simulink model "gm_gmStateSpaceHDL_uz_inverter_3ph"  (R2021b)
settings: Solver=FixedStepDiscrete  StartTime=0.0  StopTime=0.1  FixedStep=Auto  RelTol=1e-3
InitFcn:
  | load('C:\Users\valen\Documents\repos\UZ\ultrazohm_sw_working\ip_cores\uz_inverter_3ph\sschdl\uz_inverter_3ph\stateSpaceParameters.mat');
undefined symbols (not defined in the file or in its folder): udc
libraries: hdlmdlgenlib x140, dspsigops x26, simulink x17, hdlssclib x2
(part 1 of 2)
settings Model: Creator=LENOVO  LastModifiedBy=valen
settings SolverCC: AlgebraicLoopSolver=TrustRegion
settings DataIOCC: LimitDataPoints=on  SaveOutput=off  SaveTime=off
settings OptimizationCC: BlockReduction=off  ConditionallyExecuteInputs=off  DefaultParameterBehavior=Inlined  InheritOutputTypeSmallerThanSingle=on  LifeSpan=inf
settings DebuggingCC: AlgebraicLoopMsg=error  InheritedTsInSrcMsg=none  SingleTaskRateTransMsg=error  AllowSymbolicDim=off  StrictBusMsg=ErrorOnBusTreatedAsVector  SFUnexpectedBacktrackingDiag=warning  SFNoUnconditionalDefaultTransitionDiag=warning  SFExecutionAtInitializationDiag=none  SFMachineParentedDataDiag=warning  ArithmeticOperatorsInVariantConditions=warning
settings HardwareCC: ProdBitPerPointer=32  ProdBitPerSizeT=32  ProdBitPerPtrDiffT=32  ProdLargestAtomicFloat=None  ProdIntDivRoundTo=Undefined  ProdEndianess=Unspecified  ProdWordSize=32  ProdHWDeviceType=ASIC/FPGA->ASIC/FPGA  ProdEqTarget=off
settings SFSimCC: SimUseLocalCustomCode=off  CustomCodeUndefinedFunction=UseInterfaceOnly
settings RTWCC: RTWUseLocalCustomCode=off
settings CodeAppCC: StateflowObjectComments=on
settings GRTTargetCC: TargetLangStandard=C89/C90 (ANSI)
settings ConfigComp: CovScope=ReferencedModels  CovMetricSettings=dw  CovSaveCumulativeToWorkspaceVar=on  CovSaveSingleToWorkspaceVar=on  CovExternalEMLEnable=off  CovSFcnEnable=off

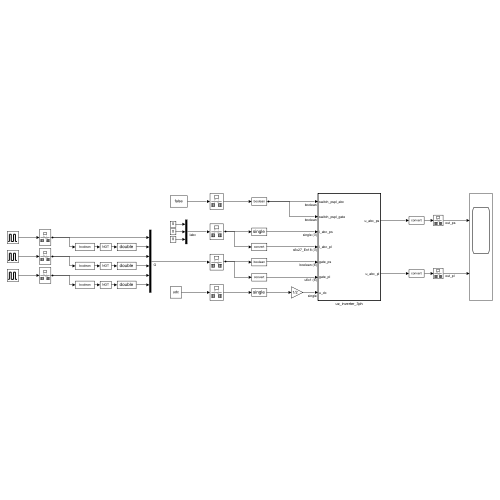
[thumbnail: Simulink's stored preview of the top-level diagram]
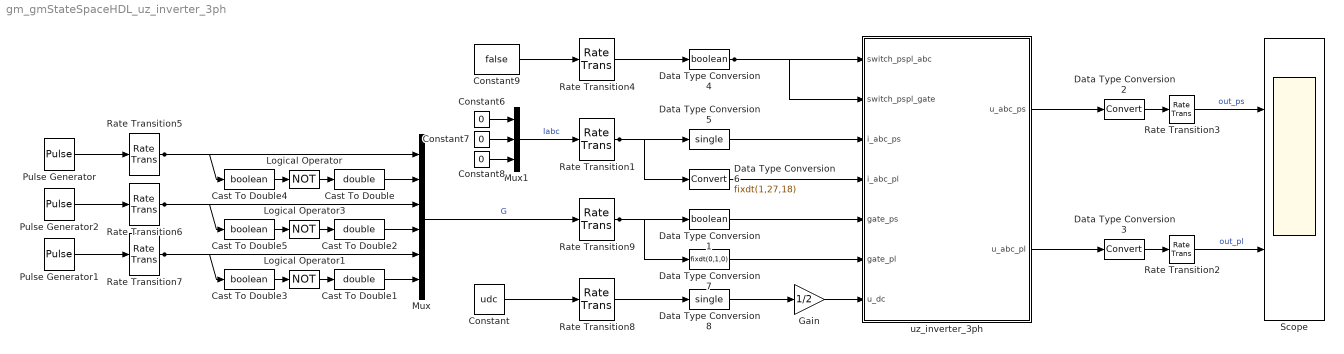
== system gm_gmStateSpaceHDL_uz_inverter_3ph ==
  Cast To Double : DataTypeConversion  OutDataTypeStr=double
  Cast To Double1 : DataTypeConversion  OutDataTypeStr=double
  Cast To Double2 : DataTypeConversion  OutDataTypeStr=double
  Cast To Double3 : DataTypeConversion  OutDataTypeStr=boolean
  Cast To Double4 : DataTypeConversion  OutDataTypeStr=boolean
  Cast To Double5 : DataTypeConversion  OutDataTypeStr=boolean
  Constant : Constant  Value=udc
  Constant6 : Constant  Value=0
  Constant7 : Constant  Value=0
  Constant8 : Constant  Value=0
  Constant9 : Constant  Value=false
  Data Type Conversion1 : DataTypeConversion  OutDataTypeStr=boolean  RndMeth=Nearest
  Data Type Conversion2 : DataTypeConversion
  Data Type Conversion3 : DataTypeConversion
  Data Type Conversion4 : DataTypeConversion  OutDataTypeStr=boolean
  Data Type Conversion5 : DataTypeConversion  OutDataTypeStr=single  RndMeth=Nearest
  Data Type Conversion6 : DataTypeConversion  OutDataTypeStr=fixdt(1,27,18)  RndMeth=Nearest
  Data Type Conversion7 : DataTypeConversion  OutDataTypeStr=fixdt(0,1,0)  RndMeth=Nearest
  Data Type Conversion8 : DataTypeConversion  OutDataTypeStr=single  RndMeth=Nearest
  Gain : Gain  Gain=1/2  OutDataTypeStr=Inherit: Same as input
  Logical Operator : Logic  Operator=NOT  AllPortsSameDT=off  OutDataTypeStr=boolean
  Logical Operator1 : Logic  Operator=NOT  AllPortsSameDT=off  OutDataTypeStr=boolean
  Logical Operator3 : Logic  Operator=NOT  AllPortsSameDT=off  OutDataTypeStr=boolean
  Mux : Mux  Inputs=6
  Mux1 : Mux  Inputs=3
  Pulse Generator : DiscretePulseGenerator  PulseType=Time based  Period=0.001  PulseWidth=50
  Pulse Generator1 : DiscretePulseGenerator  PulseType=Time based  Period=0.01  PulseWidth=50
  Pulse Generator2 : DiscretePulseGenerator  PulseType=Time based  Period=0.05  PulseWidth=50
  Rate Transition{1..9} (9 alike) : RateTransition  OutPortSampleTime=ts_inverter
  Scope : Scope  NumInputPorts=2
  uz_inverter_3ph : Subsystem  TreatAsAtomicUnit=on
  wires:
  Data Type Conversion4/1 -> uz_inverter_3ph/1(switch_pspl_abc), uz_inverter_3ph/2(switch_pspl_gate)
  Rate Transition5/1 -> Mux/1, Cast To Double4/1
  Rate Transition6/1 -> Mux/3, Cast To Double5/1
  Gain/1 -> uz_inverter_3ph/7(u_dc)
  Rate Transition8/1 -> Data Type Conversion8/1
  Constant/1 -> Rate Transition8/1
  Data Type Conversion8/1 -> Gain/1
  Rate Transition7/1 -> Mux/5, Cast To Double3/1
  Cast To Double/1 -> Mux/2
  Mux/1 -> Rate Transition9/1  "G"
  Logical Operator/1 -> Cast To Double/1
  Cast To Double1/1 -> Mux/6
  Cast To Double4/1 -> Logical Operator/1
  Cast To Double2/1 -> Mux/4
  Pulse Generator/1 -> Rate Transition5/1
  Pulse Generator2/1 -> Rate Transition6/1
  Logical Operator3/1 -> Cast To Double2/1
  Cast To Double5/1 -> Logical Operator3/1
  Pulse Generator1/1 -> Rate Transition7/1
  Cast To Double3/1 -> Logical Operator1/1
  Logical Operator1/1 -> Cast To Double1/1
  Data Type Conversion7/1 -> uz_inverter_3ph/6(gate_pl)
  Data Type Conversion5/1 -> uz_inverter_3ph/3(i_abc_ps)
  Data Type Conversion1/1 -> uz_inverter_3ph/5(gate_ps)
  Rate Transition9/1 -> Data Type Conversion1/1, Data Type Conversion7/1
  Data Type Conversion6/1 -> uz_inverter_3ph/4(i_abc_pl)
  Rate Transition1/1 -> Data Type Conversion6/1, Data Type Conversion5/1
  Constant7/1 -> Mux1/2
  Constant6/1 -> Mux1/1
  Constant8/1 -> Mux1/3
  Mux1/1 -> Rate Transition1/1  "Iabc"
  Rate Transition4/1 -> Data Type Conversion4/1
  Constant9/1 -> Rate Transition4/1
  Rate Transition2/1 -> Scope/2  "out_pl"
  Rate Transition3/1 -> Scope/1  "out_ps"
  Data Type Conversion2/1 -> Rate Transition3/1
  Data Type Conversion3/1 -> Rate Transition2/1
  uz_inverter_3ph/2(u_abc_pl) -> Data Type Conversion3/1
  uz_inverter_3ph/1(u_abc_ps) -> Data Type Conversion2/1

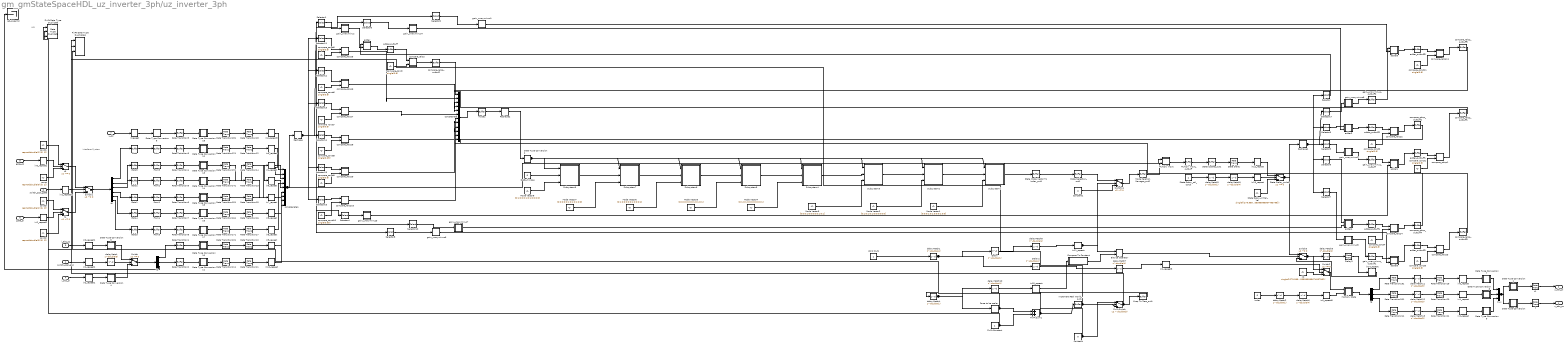
== system gm_gmStateSpaceHDL_uz_inverter_3ph/uz_inverter_3ph ==
  note: U(k)
  note: Interface System
  switch_pspl_abc : Inport  OutDataTypeStr=boolean  PortDimensions=1  SampleTime=1e-06
  switch_pspl_gate : Inport  Port=2  OutDataTypeStr=boolean  PortDimensions=1  SampleTime=1e-06
  i_abc_ps : Inport  Port=3  OutDataTypeStr=single  PortDimensions=[3]  SampleTime=1e-06
  i_abc_pl : Inport  Port=4  OutDataTypeStr=fixdt(1, 27, 18)  PortDimensions=[3]  SampleTime=1e-06
  gate_ps : Inport  Port=5  OutDataTypeStr=boolean  PortDimensions=[6]  SampleTime=1e-06  LockScale=on
  gate_pl : Inport  Port=6  OutDataTypeStr=fixdt(0, 1, 0)  PortDimensions=[6]  SampleTime=1e-06  LockScale=on
  u_dc : Inport  Port=7  OutDataTypeStr=single  PortDimensions=1  SampleTime=1e-06
  Bitwise Operator : simulink/Logic and Bit Operations/Bitwise Operator  logicop=AND  UseBitMask=off  NumInputPorts=2  BitMask=double(0)  BitMaskRealWorld=Real World Value
  Compare To Constant : Subsystem  mask(Compare To Constant){relop===, const=double(0), OutDataTypeStr=boolean, ZeroCross=on}
      mask prompts: relop "Simulink:masks:Operator_MP"; const "Simulink:masks:ConstantValue_MP"; OutDataTypeStr "Simulink:masks:OutputDataType_MP"; ZeroCross "Simulink:masks:EnableZerocrossingDetection_MP"
      mask help: Simulink:masks:CompareToConstant_MD
      mask TypeOptions relop: == | ~= | < | <= | >= | >
      mask TypeOptions OutDataTypeStr: Simulink:masks:uint8 | Simulink:masks:boolean
      mask Callback ZeroCross: sl('zeroCrossEnable', gcbh);
      mask Display: disp(str)
  Constant : Constant  Value=0  OutDataTypeStr=uint8  SampleTime=2.5e-07
  Constant1 : Constant  Value=0  OutDataTypeStr=fixdt(0, 3, 0)  SampleTime=1e-08
  Data Type Conversion : Subsystem
      mask Display: disp('NFP\nconv');
  Data Type Conversion1 : Subsystem
      mask Display: disp('NFP\nconv');
  Data Type Conversion10 : Subsystem
      mask Display: disp('NFP\nconv');
  Data Type Conversion11 : Subsystem
      mask Display: disp('NFP\nconv');
  Data Type Conversion12 : Subsystem
      mask Display: disp('NFP\nconv');
  Data Type Conversion13 : Subsystem
      mask Display: disp('NFP\nconv');
  Data Type Conversion14 : Subsystem
      mask Display: disp('NFP\nconv');
  Data Type Conversion15 : Subsystem
      mask Display: disp('NFP\nconv');
  Data Type Conversion16 : Subsystem
      mask Display: disp('NFP\nconv');
  Data Type Conversion17 : Subsystem
      mask Display: disp('NFP\nconv');
  Data Type Conversion18 : Subsystem
      mask Display: disp('NFP\nconv');
  Data Type Conversion2 : DataTypeConversion  OutDataTypeStr=boolean  SampleTime=1e-08
  Data Type Conversion3 : Subsystem
      mask Display: disp('NFP\nconv');
  Data Type Conversion4 : Subsystem
      mask Display: disp('NFP\nconv');
  Data Type Conversion6 : Subsystem
      mask Display: disp('NFP\nconv');
  Data Type Conversion7 : Subsystem
      mask Display: disp('NFP\nconv');
  Data Type Conversion8 : Subsystem
      mask Display: disp('NFP\nconv');
  Data Type Conversion9 : Subsystem
      mask Display: disp('NFP\nconv');
  Default Index : Constant  Value=0  OutDataTypeStr=fixdt(0, 3, 0)  SampleTime=1e-08
  Delay : Delay  DelayLength=double(1)  InitialCondition=0  SampleTime=2.5e-07
  Delay2 : Delay  DelayLength=double(4)  InitialCondition=0  SampleTime=2.5e-07
  Delay3 : RateTransition  OutPortSampleTimeOpt=Multiple of input port sample time  OutPortSampleTimeMultiple=25
  FixPt Constant : Constant  OutDataTypeStr=uint8  SampleTime=2.5e-07
  FixPt Data Type Duplicate : DataTypeDuplicate  DisableCoverage=on  NumInputPorts=3
  FixPt Data Type Duplicate1 : DataTypeDuplicate  DisableCoverage=on  NumInputPorts=3
  FixPt Sum1 : Sum  AccumDataTypeStr=uint8  OutDataTypeStr=uint8  SampleTime=2.5e-07
  FixPt Switch : Switch  Criteria=u2 > Threshold  Threshold=double(3)  OutDataTypeStr=uint8  SampleTime=2.5e-07
  Force to be scalar : SignalSpecification  OutDataTypeStr=uint8  Dimensions=1
  From{,1..5} (6 alike) : hdlmdlgenlib/Buffer
      settings: SourceProductBaseCode=SL
  Goto{,1..5} (6 alike) : hdlmdlgenlib/Buffer
      settings: SourceProductBaseCode=SL
  Iab_2_term2 : Terminator
  Increment Real World_out1 : hdlmdlgenlib/Buffer
      settings: SourceProductBaseCode=SL
  Index : Constant  Value=0  OutDataTypeStr=fixdt(0, 1, 0)  SampleTime=2.5e-07
  Mode Iteration Manager_out2 : hdlmdlgenlib/Buffer
      settings: SourceProductBaseCode=SL
  Mode Selection_out1 : hdlmdlgenlib/Buffer
      settings: SourceProductBaseCode=SL
  Mode Vector1 : Constant  Value=[0;0;0;1;0;1;0;0;0;1;0;0]  OutDataTypeStr=boolean  SampleTime=1e-08
  Mode Vector2 : Constant  Value=[0;1;0;1;0;1;0;0;0;0;0;0]  OutDataTypeStr=boolean  SampleTime=1e-08
  Mode Vector3 : Constant  Value=[0;0;0;1;0;0;0;0;0;1;0;1]  OutDataTypeStr=boolean  SampleTime=1e-08
  Mode Vector4 : Constant  Value=[0;1;0;1;0;0;0;0;0;0;0;1]  OutDataTypeStr=boolean  SampleTime=1e-08
  Mode Vector5 : Constant  Value=[0;0;0;0;0;0;0;1;0;1;0;1]  OutDataTypeStr=boolean  SampleTime=1e-08
  Mode Vector6 : Constant  Value=[0;1;0;0;0;0;0;1;0;0;0;1]  OutDataTypeStr=boolean  SampleTime=1e-08
  Mode Vector7 : Constant  Value=[0;0;0;0;0;1;0;1;0;1;0;0]  OutDataTypeStr=boolean  SampleTime=1e-08
  Mode Vector8 : Constant  Value=[0;1;0;0;0;1;0;1;0;0;0;0]  OutDataTypeStr=boolean  SampleTime=1e-08
  Multiply Input : Subsystem
      mask Display: disp('NFP\nSparseConstMultiply');
  Multiply Input_outbuff : hdlmdlgenlib/Buffer
      settings: SourceProductBaseCode=SL
  Multiply State : Subsystem
      mask Display: disp('NFP\nSparseConstMultiply');
  Rate Transition{1..9} (9 alike) : hdlmdlgenlib/Buffer
      settings: SourceProductBaseCode=SL
  Rate Transition{10..18} (9 alike) : RateTransition  Integrity=off  Deterministic=off  InitialCondition=double(0)  OutPortSampleTimeOpt=Multiple of input port sample time  OutPortSampleTimeMultiple=1/4
  Rate Transition{101,111,121,131,141,151,161,171,181} (9 alike) : RateTransition  OutPortSampleTimeOpt=Multiple of input port sample time  OutPortSampleTimeMultiple=100
  Rate Transition19 : RateTransition  InitialCondition=double(0)  OutPortSampleTimeOpt=Multiple of input port sample time  OutPortSampleTimeMultiple=4
  Rate Transition191 : RateTransition  OutPortSampleTimeOpt=Multiple of input port sample time  OutPortSampleTimeMultiple=25
  Rate Transition20 : RateTransition  InitialCondition=double(0)  OutPortSampleTimeOpt=Multiple of input port sample time  OutPortSampleTimeMultiple=4
  Rate Transition201 : RateTransition  OutPortSampleTimeOpt=Multiple of input port sample time  OutPortSampleTimeMultiple=25
  Rate Transition21 : RateTransition  InitialCondition=double(0)  OutPortSampleTimeOpt=Multiple of input port sample time  OutPortSampleTimeMultiple=4
  Rate Transition211 : RateTransition  OutPortSampleTimeOpt=Multiple of input port sample time  OutPortSampleTimeMultiple=25
  Reshape : Reshape  OutputDimensionality=Column vector (2-D)
  Reshape1 : Reshape  OutputDimensionality=Column vector (2-D)
  Reshape2 : Reshape
  Selector{,1..2,4,6..8,10} (8 alike) : Selector  SampleTime=1e-08  IndexOptions=Index vector (dialog)  Indices=double(1)  OutputSizes=double(0)
  Selector11 : Selector  SampleTime=1e-08  IndexOptions=Index vector (dialog)  Indices=double(2)  OutputSizes=double(0)
  Selector12 : Selector  SampleTime=1e-08  IndexOptions=Index vector (dialog)  Indices=double(3)  OutputSizes=double(0)
  Selector13 : Selector  SampleTime=1e-08  IndexOptions=Index vector (dialog)  Indices=double(4)  OutputSizes=double(0)
  Selector14 : Selector  SampleTime=1e-08  IndexOptions=Index vector (dialog)  Indices=double(5)  OutputSizes=double(0)
  Selector15 : Selector  SampleTime=1e-08  IndexOptions=Index vector (dialog)  Indices=double(6)  OutputSizes=double(0)
  Selector16 : Selector  SampleTime=1e-08  IndexOptions=Index vector (dialog)  Indices=double(7)  OutputSizes=double(0)
  Selector17 : Selector  SampleTime=1e-08  IndexOptions=Index vector (dialog)  Indices=double(2)  OutputSizes=double(0)
  Selector3 : Selector  SampleTime=1e-08  IndexOptions=Index vector (dialog)  Indices=double(3)  OutputSizes=double(0)
  Selector5 : Selector  SampleTime=1e-08  IndexOptions=Index vector (dialog)  Indices=double(2)  OutputSizes=double(0)
  Selector9 : Selector  SampleTime=1e-08  IndexOptions=Index vector (dialog)  Indices=double(3)  OutputSizes=double(0)
  State Delay : RateTransition  OutPortSampleTimeOpt=Multiple of input port sample time  OutPortSampleTimeMultiple=25
  State Delay_Initial_Val : Constant  Value=single([-279.99993896484375 -279.99993896484375 -279.99993896484375 -6.159998622301543e-10 0.0061599984765052795 -0.005599999334663153 0.0005599999567493796 -6.159998622301543e-10 0.0061599984765052795 0.0005599999567493796 0.0061599984765052795 0.0005599999567493796]).'  OutDataTypeStr=single  SampleTime=1e-08
  State Delay_ctrl_const : Constant  OutDataTypeStr=boolean  SampleTime=2.5e-07
  State Delay_switch : Switch  Criteria=u2 ~= 0  Threshold=double(0)  OutDataTypeStr=single  SampleTime=1e-08
  State Mode Vector To Index_out1 : hdlmdlgenlib/Buffer
      settings: SourceProductBaseCode=SL
  State Update_out1 : hdlmdlgenlib/Buffer
      settings: SourceProductBaseCode=SL
  Subsystem1 : Subsystem  mask{Index=fi(0,0,3,0,"hex","0")}
  Subsystem2 : Subsystem  mask{Index=fi(0,0,3,0,"hex","1")}
  Subsystem3 : Subsystem  mask{Index=fi(0,0,3,0,"hex","2")}
  Subsystem4 : Subsystem  mask{Index=fi(0,0,3,0,"hex","3")}
  Subsystem5 : Subsystem  mask{Index=fi(0,0,3,0,"hex","4")}
  Subsystem6 : Subsystem  mask{Index=fi(0,0,3,0,"hex","5")}
  Subsystem7 : Subsystem  mask{Index=fi(0,0,3,0,"hex","6")}
  Subsystem8 : Subsystem  mask{Index=fi(0,0,3,0,"hex","7")}
  Switch : Switch  Criteria=u2 ~= 0  Threshold=double(0)  OutDataTypeStr=double  SampleTime=1e-08
  Switch1 : Switch  Criteria=u2 ~= 0  Threshold=double(0)  OutDataTypeStr=double  SampleTime=1e-08
  Switch11 : Switch  Criteria=u2 ~= 0  Threshold=double(0)  OutDataTypeStr=fixdt(0, 3, 0)  SampleTime=1e-08
  Switch2 : Switch  Criteria=u2 ~= 0  Threshold=double(0)  OutDataTypeStr=single  SampleTime=1e-08
  Switch3 : Switch  Criteria=u2 ~= 0  Threshold=double(0)  OutDataTypeStr=single  SampleTime=1e-08
  Valid Out1 : Constant  OutDataTypeStr=boolean  SampleTime=2.5e-07
  Wrap To Zero_out1 : hdlmdlgenlib/Buffer
      settings: SourceProductBaseCode=SL
  X0 : Constant  Value=single([-279.99993896484375 -279.99993896484375 -279.99993896484375 -6.159998622301543e-10 0.0061599984765052795 -0.005599999334663153 0.0005599999567493796 -6.159998622301543e-10 0.0061599984765052795 0.0005599999567493796 0.0061599984765052795 0.0005599999567493796]).'  OutDataTypeStr=single  SampleTime=1e-08
  adder : Subsystem
      mask Display: disp('NFP\nadd');
  adder1 : Subsystem
      mask Display: disp('NFP\nadd');
  adder2 : Subsystem
      mask Display: disp('NFP\nadd');
  adder3 : Subsystem
      mask Display: disp('NFP\nadd');
  adder4 : Subsystem
      mask Display: disp('NFP\nadd');
  adder5 : Subsystem
      mask Display: disp('NFP\nadd');
  adder_outbuff{,1..5} (6 alike) : hdlmdlgenlib/Buffer
      settings: SourceProductBaseCode=SL
  compare_const{,1..4,11} (6 alike) : Constant  Value=single(0.8)  OutDataTypeStr=single  SampleTime=1e-08
  compare_const10 : Constant  Value=single(0.05)  OutDataTypeStr=single  SampleTime=1e-08
  compare_const{5..7,9} (4 alike) : Constant  Value=single(0.5)  OutDataTypeStr=single  SampleTime=1e-08
  compare_const8 : Constant  Value=single(0.05)  OutDataTypeStr=single  SampleTime=1e-08
  compare_relop : Subsystem
      mask Display: disp('NFP\nrelop');
  compare_relop1 : Subsystem
      mask Display: disp('NFP\nrelop');
  compare_relop10 : Subsystem
      mask Display: disp('NFP\nrelop');
  compare_relop11 : Subsystem
      mask Display: disp('NFP\nrelop');
  compare_relop2 : Subsystem
      mask Display: disp('NFP\nrelop');
  compare_relop3 : Subsystem
      mask Display: disp('NFP\nrelop');
  compare_relop4 : Subsystem
      mask Display: disp('NFP\nrelop');
  compare_relop5 : Subsystem
      mask Display: disp('NFP\nrelop');
  compare_relop6 : Subsystem
      mask Display: disp('NFP\nrelop');
  compare_relop7 : Subsystem
      mask Display: disp('NFP\nrelop');
  compare_relop8 : Subsystem
      mask Display: disp('NFP\nrelop');
  compare_relop9 : Subsystem
      mask Display: disp('NFP\nrelop');
  compare_relop_outbuff{,1..5} (6 alike) : hdlmdlgenlib/Buffer
      settings: SourceProductBaseCode=SL
  concatenate : Concatenate  NumInputs=12  ConcatenateDimension=2
  concatenate1 : Concatenate  NumInputs=9
  const : Constant  Value="repmat(double(0),[6  1])"  OutDataTypeStr=double  SampleTime=1e-08
  const1 : Constant  Value="repmat(double(1),[6  1])"  OutDataTypeStr=double  SampleTime=1e-08
  const2 : Constant  Value="repmat(double(0),[6  1])"  OutDataTypeStr=double  SampleTime=1e-08
  const3 : Constant  Value="repmat(double(1),[6  1])"  OutDataTypeStr=double  SampleTime=1e-08
  delayMatch : Delay  DelayLength=double(3)  InitialCondition=0  SampleTime=1e-08
  delayMatch{1,6..10} (6 alike) : Delay  DelayLength=double(4)  InitialCondition=0  SampleTime=2.5e-07
  delayMatch11 : Delay  DelayLength=double(3)  InitialCondition=0  SampleTime=2.5e-07
  delayMatch12 : Delay  DelayLength=double(3)  InitialCondition=0  SampleTime=2.5e-07
  delayMatch13 : Delay  DelayLength=double(3)  InitialCondition=0  SampleTime=2.5e-07
  delayMatch2 : Delay  DelayLength=double(1)  InitialCondition=0  SampleTime=2.5e-07
  delayMatch3 : Delay  DelayLength=double(1)  InitialCondition=0  SampleTime=2.5e-07
  delayMatch4 : Delay  DelayLength=double(1)  InitialCondition=0  SampleTime=2.5e-07
  delayMatch5 : Delay  DelayLength=double(1)  InitialCondition=0  SampleTime=1e-08
  gain_unaryminus : Subsystem
      mask Display: disp('NFP\numinus');
  gain_unaryminus1 : Subsystem
      mask Display: disp('NFP\numinus');
  gain_unaryminus2 : Subsystem
      mask Display: disp('NFP\numinus');
  gain_unaryminus3 : Subsystem
      mask Display: disp('NFP\numinus');
  gain_unaryminus4 : Subsystem
      mask Display: disp('NFP\numinus');
  gain_unaryminus5 : Subsystem
      mask Display: disp('NFP\numinus');
  gain_unaryminus6 : Subsystem
      mask Display: disp('NFP\numinus');
  gain_unaryminus7 : Subsystem
      mask Display: disp('NFP\numinus');
  gain_unaryminus8 : Subsystem
      mask Display: disp('NFP\numinus');
  gain_unaryminus_outbuff : hdlmdlgenlib/Buffer
      settings: SourceProductBaseCode=SL
  gain_unaryminus_outbuff1 : hdlmdlgenlib/Buffer
      settings: SourceProductBaseCode=SL
  gain_unaryminus_outbuff2 : hdlmdlgenlib/Buffer
      settings: SourceProductBaseCode=SL
  in0_repeat : dspsigops/Repeat  N=double(100)  RateOptions=Allow multirate processing  ic=0  mode=Unused parameter value
  in0_repeat1 : dspsigops/Repeat  N=double(100)  RateOptions=Allow multirate processing  ic=0  mode=Unused parameter value
  in0_repeat2 : dspsigops/Repeat  N=double(100)  RateOptions=Allow multirate processing  ic=0  mode=Unused parameter value
  in0_repeat3 : dspsigops/Repeat  N=double(25)  RateOptions=Allow multirate processing  ic=0  mode=Unused parameter value
  in10_repeat : dspsigops/Repeat  N=double(25)  RateOptions=Allow multirate processing  ic=0  mode=Unused parameter value
  in11_repeat : dspsigops/Repeat  N=double(25)  RateOptions=Allow multirate processing  ic=0  mode=Unused parameter value
  in12_repeat : dspsigops/Repeat  N=double(25)  RateOptions=Allow multirate processing  ic=0  mode=Unused parameter value
  in13_repeat : dspsigops/Repeat  N=double(25)  RateOptions=Allow multirate processing  ic=0  mode=Unused parameter value
  in14_repeat : dspsigops/Repeat  N=double(25)  RateOptions=Allow multirate processing  ic=0  mode=Unused parameter value
  in15_repeat : dspsigops/Repeat  N=double(25)  RateOptions=Allow multirate processing  ic=0  mode=Unused parameter value
  in1_repeat : dspsigops/Repeat  N=double(100)  RateOptions=Allow multirate processing  ic=0  mode=Unused parameter value
  in1_repeat1 : dspsigops/Repeat  N=double(100)  RateOptions=Allow multirate processing  ic=0  mode=Unused parameter value
  in1_repeat2 : dspsigops/Repeat  N=double(100)  RateOptions=Allow multirate processing  ic=0  mode=Unused parameter value
  in1_repeat3 : dspsigops/Repeat  N=double(25)  RateOptions=Allow multirate processing  ic=0  mode=Unused parameter value
  in2_repeat : dspsigops/Repeat  N=double(100)  RateOptions=Allow multirate processing  ic=0  mode=Unused parameter value
  in2_repeat1 : dspsigops/Repeat  N=double(100)  RateOptions=Allow multirate processing  ic=0  mode=Unused parameter value
  in2_repeat2 : dspsigops/Repeat  N=double(100)  RateOptions=Allow multirate processing  ic=0  mode=Unused parameter value
  in2_repeat3 : dspsigops/Repeat  N=double(25)  RateOptions=Allow multirate processing  ic=0  mode=Unused parameter value
  in3_repeat : dspsigops/Repeat  N=double(25)  RateOptions=Allow multirate processing  ic=0  mode=Unused parameter value
  in4_repeat : dspsigops/Repeat  N=double(25)  RateOptions=Allow multirate processing  ic=0  mode=Unused parameter value
  in5_repeat : dspsigops/Repeat  N=double(25)  RateOptions=Allow multirate processing  ic=0  mode=Unused parameter value
  in6_repeat : dspsigops/Repeat  N=double(25)  RateOptions=Allow multirate processing  ic=0  mode=Unused parameter value
  in7_repeat : dspsigops/Repeat  N=double(25)  RateOptions=Allow multirate processing  ic=0  mode=Unused parameter value
  in8_repeat : dspsigops/Repeat  N=double(25)  RateOptions=Allow multirate processing  ic=0  mode=Unused parameter value
  in9_repeat : dspsigops/Repeat  N=double(25)  RateOptions=Allow multirate processing  ic=0  mode=Unused parameter value
  inrepeat : dspsigops/Repeat  N=double(100)  RateOptions=Allow multirate processing  ic=0  mode=Unused parameter value
  modes : hdlmdlgenlib/Buffer
      settings: SourceProductBaseCode=SL
  mux : Mux  Inputs=3
  t : RateTransition  OutPortSampleTimeOpt=Multiple of input port sample time  OutPortSampleTimeMultiple=100
  t1 : RateTransition  OutPortSampleTimeOpt=Multiple of input port sample time  OutPortSampleTimeMultiple=100
  t2 : Demux  Outputs=3
  t3 : Switch  Criteria=u2 ~= 0  Threshold=double(0)  OutDataTypeStr=double  SampleTime=1e-08
  t4 : Switch  Criteria=u2 ~= 0  Threshold=double(0)  OutDataTypeStr=double  SampleTime=1e-08
  t5 : Demux  Outputs=6
  t6 : Demux  Outputs=3
  u_abc_ps : Outport  SampleTime=1e-06
  u_abc_pl : Outport  Port=2  SampleTime=1e-06
  wires:
  switch_pspl_abc/1 -> in1_repeat1/1
  switch_pspl_gate/1 -> in1_repeat2/1
  i_abc_ps/1 -> in0_repeat1/1
  i_abc_pl/1 -> in2_repeat1/1
  gate_ps/1 -> in0_repeat2/1
  gate_pl/1 -> in2_repeat2/1
  u_dc/1 -> inrepeat/1
  Rate Transition10/1 -> in9_repeat/1
  Rate Transition11/1 -> in10_repeat/1
  Rate Transition12/1 -> in3_repeat/1
  Rate Transition13/1 -> in7_repeat/1
  Rate Transition14/1 -> in6_repeat/1
  Rate Transition15/1 -> in4_repeat/1
  Rate Transition16/1 -> in8_repeat/1
  Rate Transition17/1 -> in5_repeat/1
  Rate Transition18/1 -> in2_repeat3/1
  Rate Transition19/1 -> in0_repeat/1
  Rate Transition20/1 -> in1_repeat/1
  Rate Transition21/1 -> in2_repeat/1
  delayMatch6/1 -> in0_repeat3/1
  delayMatch8/1 -> in11_repeat/1
  delayMatch7/1 -> in1_repeat3/1
  delayMatch1/1 -> Delay2/1, Delay/1
  delayMatch10/1 -> in15_repeat/1
  delayMatch9/1 -> in13_repeat/1
  delayMatch11/1 -> Rate Transition19/1
  delayMatch12/1 -> Rate Transition20/1
  delayMatch13/1 -> Rate Transition21/1
  t/1 -> u_abc_ps/1
  t1/1 -> u_abc_pl/1
  Rate Transition101/1 -> Rate Transition10/1
  Rate Transition111/1 -> Rate Transition11/1
  Rate Transition121/1 -> Rate Transition12/1
  Rate Transition131/1 -> Rate Transition13/1
  Rate Transition141/1 -> Rate Transition14/1
  Rate Transition151/1 -> Rate Transition15/1
  Rate Transition161/1 -> Rate Transition16/1
  Rate Transition171/1 -> Rate Transition17/1
  Rate Transition181/1 -> Rate Transition18/1
  delayMatch2/1 -> delayMatch6/1
  Delay2/1 -> delayMatch7/1
  Delay/1 -> delayMatch8/1
  delayMatch3/1 -> delayMatch9/1
  delayMatch4/1 -> delayMatch10/1, Force to be scalar/1
  Delay3/1 -> in14_repeat/1
  State Delay/1 -> in12_repeat/1
  Rate Transition191/1 -> delayMatch11/1
  Rate Transition201/1 -> delayMatch12/1
  Rate Transition211/1 -> delayMatch13/1
  Data Type Conversion/1(Out1) -> t/1
  Data Type Conversion1/1(Out1) -> t1/1
  in0_repeat/1 -> Data Type Conversion7/1(In1)
  in1_repeat/1 -> Data Type Conversion8/1(In1)
  in2_repeat/1 -> Data Type Conversion9/1(In1)
  mux/1 -> Data Type Conversion/1(In1), Data Type Conversion1/1(In1)
  Data Type Conversion7/1(Out1) -> mux/1
  Data Type Conversion8/1(Out1) -> mux/2
  Data Type Conversion9/1(Out1) -> mux/3
  Data Type Conversion10/1(Out1) -> Rate Transition101/1
  Data Type Conversion11/1(Out1) -> Rate Transition111/1
  in0_repeat1/1 -> Data Type Conversion3/1(In1)
  in1_repeat1/1 -> delayMatch/1
  in2_repeat1/1 -> Data Type Conversion4/1(In1)
  Rate Transition2/1 -> Data Type Conversion11/1(In1)
  Switch/1 -> t2/1
  Rate Transition1/1 -> Data Type Conversion10/1(In1)
  t2/1 -> Rate Transition1/1
  t2/2 -> Rate Transition2/1
  t2/3 -> Iab_2_term2/1
  delayMatch/1 -> Switch/2
  Data Type Conversion3/1(Out1) -> Switch/1
  Data Type Conversion4/1(Out1) -> Switch/3
  Data Type Conversion12/1(Out1) -> Rate Transition121/1
  Data Type Conversion13/1(Out1) -> Rate Transition131/1
  Data Type Conversion14/1(Out1) -> Rate Transition141/1
  Data Type Conversion15/1(Out1) -> Rate Transition151/1
  Data Type Conversion16/1(Out1) -> Rate Transition161/1
  Data Type Conversion17/1(Out1) -> Rate Transition171/1
  in0_repeat2/1 -> t3/2
  in1_repeat2/1 -> Switch1/2
  in2_repeat2/1 -> t4/2
  Rate Transition4/1 -> Data Type Conversion13/1(In1)
  From5/1 -> Rate Transition4/1
  Goto5/1 -> From5/1
  Rate Transition5/1 -> Data Type Conversion14/1(In1)
  From2/1 -> Rate Transition5/1
  Goto2/1 -> From2/1
  Rate Transition6/1 -> Data Type Conversion15/1(In1)
  From1/1 -> Rate Transition6/1
  Goto1/1 -> From1/1
  Rate Transition7/1 -> Data Type Conversion16/1(In1)
  From4/1 -> Rate Transition7/1
  Goto4/1 -> From4/1
  Rate Transition8/1 -> Data Type Conversion17/1(In1)
  From3/1 -> Rate Transition8/1
  Goto3/1 -> From3/1
  t3/1 -> Switch1/1
  t4/1 -> Switch1/3
  Switch1/1 -> t5/1
  Goto/1 -> From/1
  From/1 -> Rate Transition3/1
  Rate Transition3/1 -> Data Type Conversion12/1(In1)
  const/1 -> t3/3
  const1/1 -> t3/1
  const2/1 -> t4/3
  const3/1 -> t4/1
  t5/1 -> Goto/1
  t5/2 -> Goto5/1
  t5/3 -> Goto2/1
  t5/4 -> Goto1/1
  t5/5 -> Goto4/1
  t5/6 -> Goto3/1
  Data Type Conversion18/1(Out1) -> Rate Transition181/1
  inrepeat/1 -> Data Type Conversion6/1(In1)
  Rate Transition9/1 -> Data Type Conversion18/1(In1)
  Data Type Conversion6/1(Out1) -> Rate Transition9/1
  Valid Out1/1 -> delayMatch1/1
  Index/1 -> delayMatch2/1
  State Delay_ctrl_const/1 -> delayMatch3/1
  Constant/1 -> FixPt Switch/1, FixPt Data Type Duplicate1/3
  FixPt Switch/1 -> Wrap To Zero_out1/1, FixPt Data Type Duplicate1/1
  Increment Real World_out1/1 -> FixPt Switch/3, FixPt Switch/2, FixPt Data Type Duplicate1/2
  Force to be scalar/1 -> FixPt Sum1/1, FixPt Data Type Duplicate/2
  FixPt Constant/1 -> FixPt Sum1/2, FixPt Data Type Duplicate/3
  FixPt Sum1/1 -> Increment Real World_out1/1, FixPt Data Type Duplicate/1
  Wrap To Zero_out1/1 -> delayMatch4/1
  delayMatch5/1 -> Delay3/1
  State Update_out1/1 -> State Delay/1
  in0_repeat3/1 -> Multiply State/2(In2)
  in1_repeat3/1 -> Switch2/2
  in2_repeat3/1 -> concatenate1/1
  in3_repeat/1 -> concatenate1/2
  in4_repeat/1 -> concatenate1/3
  in5_repeat/1 -> concatenate1/4
  in6_repeat/1 -> concatenate1/5
  in7_repeat/1 -> concatenate1/6
  in8_repeat/1 -> concatenate1/7
  in9_repeat/1 -> concatenate1/8
  in10_repeat/1 -> concatenate1/9
  in11_repeat/1 -> Bitwise Operator/1, Switch11/2
  in12_repeat/1 -> State Delay_switch/1
  in13_repeat/1 -> State Delay_switch/2
  in14_repeat/1 -> Switch3/3
  in15_repeat/1 -> Compare To Constant/1(u)
  X0/1 -> Switch2/3
  Switch2/1 -> Multiply State/1(In1)
  compare_const/1 -> compare_relop/2(In2)
  compare_relop_outbuff/1 -> concatenate/1
  Selector/1 -> adder/1(In1)
  adder_outbuff/1 -> compare_relop/1(In1)
  Selector1/1 -> gain_unaryminus/1(In1)
  Selector2/1 -> gain_unaryminus1/1(In1)
  compare_const1/1 -> compare_relop1/2(In2)
  compare_relop_outbuff1/1 -> concatenate/5
  Selector3/1 -> gain_unaryminus2/1(In1)
  gain_unaryminus_outbuff/1 -> adder1/1(In1)
  adder_outbuff1/1 -> compare_relop1/1(In1)
  Selector4/1 -> gain_unaryminus3/1(In1)
  compare_const2/1 -> compare_relop2/2(In2)
  compare_relop_outbuff2/1 -> concatenate/7
  Selector5/1 -> adder2/1(In1)
  adder_outbuff2/1 -> compare_relop2/1(In1)
  Selector6/1 -> gain_unaryminus4/1(In1)
  compare_const3/1 -> compare_relop3/2(In2)
  compare_relop_outbuff3/1 -> concatenate/9
  Selector7/1 -> gain_unaryminus5/1(In1)
  gain_unaryminus_outbuff1/1 -> adder3/1(In1)
  adder_outbuff3/1 -> compare_relop3/1(In1)
  Selector8/1 -> gain_unaryminus6/1(In1)
  compare_const4/1 -> compare_relop4/2(In2)
  compare_relop_outbuff4/1 -> concatenate/11
  Selector9/1 -> adder4/1(In1)
  adder_outbuff4/1 -> compare_relop4/1(In1)
  Selector10/1 -> gain_unaryminus7/1(In1)
  compare_const5/1 -> compare_relop5/2(In2)
  Selector11/1 -> compare_relop5/1(In1)
  compare_const6/1 -> compare_relop6/2(In2)
  Selector12/1 -> compare_relop6/1(In1)
  compare_const7/1 -> compare_relop7/2(In2)
  Selector13/1 -> compare_relop7/1(In1)
  compare_const8/1 -> compare_relop8/2(In2)
  Selector14/1 -> compare_relop8/1(In1)
  compare_const9/1 -> compare_relop9/2(In2)
  Selector15/1 -> compare_relop9/1(In1)
  compare_const10/1 -> compare_relop10/2(In2)
  Selector16/1 -> compare_relop10/1(In1)
  Reshape/1 -> Selector1/1, Selector2/1, Selector4/1, Selector6/1, Selector8/1, Selector10/1, Selector11/1, Selector12/1, Selector13/1, Selector14/1, Selector15/1, Selector16/1
  Multiply Input_outbuff/1 -> State Update_out1/1
  Mode Iteration Manager_out2/1 -> Multiply Input/2(In2)
  Constant1/1 -> Switch11/3
  Switch11/1 -> Mode Iteration Manager_out2/1
  Mode Selection_out1/1 -> Switch11/1
  State Mode Vector To Index_out1/1 -> Mode Selection_out1/1
  Default Index/1 -> Subsystem8/2(In2)
  Mode Vector8/1 -> Subsystem8/3(In3)
  Subsystem8/1(Out1) -> Subsystem7/2(In2)
  Mode Vector7/1 -> Subsystem7/3(In3)
  Subsystem7/1(Out1) -> Subsystem6/2(In2)
  Mode Vector6/1 -> Subsystem6/3(In3)
  Subsystem6/1(Out1) -> Subsystem5/2(In2)
  Mode Vector5/1 -> Subsystem5/3(In3)
  Subsystem5/1(Out1) -> Subsystem4/2(In2)
  Mode Vector4/1 -> Subsystem4/3(In3)
  Subsystem4/1(Out1) -> Subsystem3/2(In2)
  Mode Vector3/1 -> Subsystem3/3(In3)
  Subsystem3/1(Out1) -> Subsystem2/2(In2)
  Mode Vector2/1 -> Subsystem2/3(In3)
  Subsystem2/1(Out1) -> Subsystem1/2(In2)
  Mode Vector1/1 -> Subsystem1/3(In3)
  Subsystem1/1(Out1) -> State Mode Vector To Index_out1/1
  Data Type Conversion2/1 -> Subsystem1/1(In1), Subsystem2/1(In1), Subsystem3/1(In1), Subsystem4/1(In1), Subsystem5/1(In1), Subsystem6/1(In1), Subsystem7/1(In1), Subsystem8/1(In1)
  Reshape2/1 -> Data Type Conversion2/1
  modes/1 -> Reshape2/1
  concatenate/1 -> modes/1
  compare_const11/1 -> compare_relop11/2(In2)
  compare_relop_outbuff5/1 -> concatenate/3
  adder_outbuff5/1 -> compare_relop11/1(In1)
  gain_unaryminus_outbuff2/1 -> adder5/1(In1)
  Selector17/1 -> gain_unaryminus8/1(In1)
  Reshape1/1 -> Selector17/1, Selector3/1, Selector7/1, Selector/1, Selector5/1, Selector9/1
  State Delay_Initial_Val/1 -> State Delay_switch/3
  State Delay_switch/1 -> Switch3/1, Reshape1/1
  Compare To Constant/1(y) -> Bitwise Operator/2
  Bitwise Operator/1 -> Switch3/2
  t6/1 -> Rate Transition191/1
  t6/2 -> Rate Transition201/1
  t6/3 -> Rate Transition211/1
  compare_relop/1(Out1) -> compare_relop_outbuff/1
  adder/1(Out1) -> adder_outbuff/1
  gain_unaryminus/1(Out1) -> adder/2(In2)
  gain_unaryminus1/1(Out1) -> adder5/2(In2)
  compare_relop1/1(Out1) -> compare_relop_outbuff1/1
  gain_unaryminus2/1(Out1) -> gain_unaryminus_outbuff/1
  adder1/1(Out1) -> adder_outbuff1/1
  gain_unaryminus3/1(Out1) -> adder1/2(In2)
  compare_relop2/1(Out1) -> compare_relop_outbuff2/1
  adder2/1(Out1) -> adder_outbuff2/1
  gain_unaryminus4/1(Out1) -> adder2/2(In2)
  compare_relop3/1(Out1) -> compare_relop_outbuff3/1
  gain_unaryminus5/1(Out1) -> gain_unaryminus_outbuff1/1
  adder3/1(Out1) -> adder_outbuff3/1
  gain_unaryminus6/1(Out1) -> adder3/2(In2)
  compare_relop4/1(Out1) -> compare_relop_outbuff4/1
  adder4/1(Out1) -> adder_outbuff4/1
  gain_unaryminus7/1(Out1) -> adder4/2(In2)
  compare_relop5/1(Out1) -> concatenate/2
  compare_relop6/1(Out1) -> concatenate/4
  compare_relop7/1(Out1) -> concatenate/6
  compare_relop8/1(Out1) -> concatenate/8
  compare_relop9/1(Out1) -> concatenate/10
  compare_relop10/1(Out1) -> concatenate/12
  compare_relop11/1(Out1) -> compare_relop_outbuff5/1
  adder5/1(Out1) -> adder_outbuff5/1
  gain_unaryminus8/1(Out1) -> gain_unaryminus_outbuff2/1
  Multiply State/1(Out1) -> t6/1
  Multiply Input/1(Out1) -> Multiply Input_outbuff/1
  concatenate1/1 -> Reshape/1, Multiply Input/1(In1)
  Switch3/1 -> delayMatch5/1, Switch2/1

== system gm_gmStateSpaceHDL_uz_inverter_3ph/uz_inverter_3ph/Compare To Constant ==
  u : Inport  OutDataTypeStr=uint8  SampleTime=1e-08
  Compare : RelationalOperator  Operator===  OutDataTypeStr=boolean  SampleTime=1e-08  RndMeth=Nearest  InputSameDT=on
  Constant : Constant  Value=fi(0,0,8,0,'int',0)  OutDataTypeStr=fixdt(0, 8, 0)  SampleTime=1e-08
  y : Outport  SampleTime=1e-08
  wires:
  Compare/1 -> y/1
  Constant/1 -> Compare/2
  u/1 -> Compare/1

== system gm_gmStateSpaceHDL_uz_inverter_3ph/uz_inverter_3ph/Data Type Conversion ==
  In1 : Inport
  Data Type Conversion : DataTypeConversion  OutDataTypeStr=single  RndMeth=Nearest  SampleTime=1e-08
  Data Type Conversion_pd1 : Delay  DelayLength=3
  Out1 : Outport
  wires:
  In1/1 -> Data Type Conversion/1
  Data Type Conversion/1 -> Data Type Conversion_pd1/1
  Data Type Conversion_pd1/1 -> Out1/1

== system gm_gmStateSpaceHDL_uz_inverter_3ph/uz_inverter_3ph/Data Type Conversion1 ==
  In1 : Inport
  Data Type Conversion1 : DataTypeConversion  OutDataTypeStr=fixdt(1, 27, 16)  RndMeth=Nearest  SampleTime=1e-08
  Data Type Conversion1_pd1 : Delay  DelayLength=3
  Out1 : Outport
  wires:
  In1/1 -> Data Type Conversion1/1
  Data Type Conversion1/1 -> Data Type Conversion1_pd1/1
  Data Type Conversion1_pd1/1 -> Out1/1

== system gm_gmStateSpaceHDL_uz_inverter_3ph/uz_inverter_3ph/Data Type Conversion10 ==
  In1 : Inport
  Data Type Conversion10 : DataTypeConversion  OutDataTypeStr=single  RndMeth=Nearest  SampleTime=1e-08
  Data Type Conversion10_pd1 : Delay  DelayLength=3
  Out1 : Outport
  wires:
  In1/1 -> Data Type Conversion10/1
  Data Type Conversion10/1 -> Data Type Conversion10_pd1/1
  Data Type Conversion10_pd1/1 -> Out1/1

== system gm_gmStateSpaceHDL_uz_inverter_3ph/uz_inverter_3ph/Data Type Conversion11 ==
  In1 : Inport
  Data Type Conversion11 : DataTypeConversion  OutDataTypeStr=single  RndMeth=Nearest  SampleTime=1e-08
  Data Type Conversion11_pd1 : Delay  DelayLength=3
  Out1 : Outport
  wires:
  In1/1 -> Data Type Conversion11/1
  Data Type Conversion11/1 -> Data Type Conversion11_pd1/1
  Data Type Conversion11_pd1/1 -> Out1/1

== system gm_gmStateSpaceHDL_uz_inverter_3ph/uz_inverter_3ph/Data Type Conversion12 ==
  In1 : Inport
  Data Type Conversion12 : DataTypeConversion  OutDataTypeStr=single  RndMeth=Nearest  SampleTime=1e-08
  Data Type Conversion12_pd1 : Delay  DelayLength=3
  Out1 : Outport
  wires:
  In1/1 -> Data Type Conversion12/1
  Data Type Conversion12/1 -> Data Type Conversion12_pd1/1
  Data Type Conversion12_pd1/1 -> Out1/1

== system gm_gmStateSpaceHDL_uz_inverter_3ph/uz_inverter_3ph/Data Type Conversion13 ==
  In1 : Inport
  Data Type Conversion13 : DataTypeConversion  OutDataTypeStr=single  RndMeth=Nearest  SampleTime=1e-08
  Data Type Conversion13_pd1 : Delay  DelayLength=3
  Out1 : Outport
  wires:
  In1/1 -> Data Type Conversion13/1
  Data Type Conversion13/1 -> Data Type Conversion13_pd1/1
  Data Type Conversion13_pd1/1 -> Out1/1

== system gm_gmStateSpaceHDL_uz_inverter_3ph/uz_inverter_3ph/Data Type Conversion14 ==
  In1 : Inport
  Data Type Conversion14 : DataTypeConversion  OutDataTypeStr=single  RndMeth=Nearest  SampleTime=1e-08
  Data Type Conversion14_pd1 : Delay  DelayLength=3
  Out1 : Outport
  wires:
  In1/1 -> Data Type Conversion14/1
  Data Type Conversion14/1 -> Data Type Conversion14_pd1/1
  Data Type Conversion14_pd1/1 -> Out1/1

== system gm_gmStateSpaceHDL_uz_inverter_3ph/uz_inverter_3ph/Data Type Conversion15 ==
  In1 : Inport
  Data Type Conversion15 : DataTypeConversion  OutDataTypeStr=single  RndMeth=Nearest  SampleTime=1e-08
  Data Type Conversion15_pd1 : Delay  DelayLength=3
  Out1 : Outport
  wires:
  In1/1 -> Data Type Conversion15/1
  Data Type Conversion15/1 -> Data Type Conversion15_pd1/1
  Data Type Conversion15_pd1/1 -> Out1/1

== system gm_gmStateSpaceHDL_uz_inverter_3ph/uz_inverter_3ph/Data Type Conversion16 ==
  In1 : Inport
  Data Type Conversion16 : DataTypeConversion  OutDataTypeStr=single  RndMeth=Nearest  SampleTime=1e-08
  Data Type Conversion16_pd1 : Delay  DelayLength=3
  Out1 : Outport
  wires:
  In1/1 -> Data Type Conversion16/1
  Data Type Conversion16/1 -> Data Type Conversion16_pd1/1
  Data Type Conversion16_pd1/1 -> Out1/1

== system gm_gmStateSpaceHDL_uz_inverter_3ph/uz_inverter_3ph/Data Type Conversion17 ==
  In1 : Inport
  Data Type Conversion17 : DataTypeConversion  OutDataTypeStr=single  RndMeth=Nearest  SampleTime=1e-08
  Data Type Conversion17_pd1 : Delay  DelayLength=3
  Out1 : Outport
  wires:
  In1/1 -> Data Type Conversion17/1
  Data Type Conversion17/1 -> Data Type Conversion17_pd1/1
  Data Type Conversion17_pd1/1 -> Out1/1

== system gm_gmStateSpaceHDL_uz_inverter_3ph/uz_inverter_3ph/Data Type Conversion18 ==
  In1 : Inport
  Data Type Conversion18 : DataTypeConversion  OutDataTypeStr=single  RndMeth=Nearest  SampleTime=1e-08
  Data Type Conversion18_pd1 : Delay  DelayLength=3
  Out1 : Outport
  wires:
  In1/1 -> Data Type Conversion18/1
  Data Type Conversion18/1 -> Data Type Conversion18_pd1/1
  Data Type Conversion18_pd1/1 -> Out1/1

== system gm_gmStateSpaceHDL_uz_inverter_3ph/uz_inverter_3ph/Data Type Conversion3 ==
  In1 : Inport
  Data Type Conversion3 : DataTypeConversion  OutDataTypeStr=double  RndMeth=Nearest  SampleTime=1e-08
  Data Type Conversion3_pd1 : Delay  DelayLength=3
  Out1 : Outport
  wires:
  In1/1 -> Data Type Conversion3/1
  Data Type Conversion3/1 -> Data Type Conversion3_pd1/1
  Data Type Conversion3_pd1/1 -> Out1/1

== system gm_gmStateSpaceHDL_uz_inverter_3ph/uz_inverter_3ph/Data Type Conversion4 ==
  In1 : Inport
  Data Type Conversion4 : DataTypeConversion  OutDataTypeStr=double  RndMeth=Nearest  SampleTime=1e-08
  Data Type Conversion4_pd1 : Delay  DelayLength=3
  Out1 : Outport
  wires:
  In1/1 -> Data Type Conversion4/1
  Data Type Conversion4/1 -> Data Type Conversion4_pd1/1
  Data Type Conversion4_pd1/1 -> Out1/1

== system gm_gmStateSpaceHDL_uz_inverter_3ph/uz_inverter_3ph/Data Type Conversion6 ==
  In1 : Inport
  Data Type Conversion6 : DataTypeConversion  OutDataTypeStr=double  RndMeth=Nearest  SampleTime=1e-08
  Data Type Conversion6_pd1 : Delay  DelayLength=3
  Out1 : Outport
  wires:
  In1/1 -> Data Type Conversion6/1
  Data Type Conversion6/1 -> Data Type Conversion6_pd1/1
  Data Type Conversion6_pd1/1 -> Out1/1

== system gm_gmStateSpaceHDL_uz_inverter_3ph/uz_inverter_3ph/Data Type Conversion7 ==
  In1 : Inport
  Data Type Conversion7 : DataTypeConversion  OutDataTypeStr=double  RndMeth=Nearest  SampleTime=1e-08
  Data Type Conversion7_pd1 : Delay  DelayLength=3
  Out1 : Outport
  wires:
  In1/1 -> Data Type Conversion7/1
  Data Type Conversion7/1 -> Data Type Conversion7_pd1/1
  Data Type Conversion7_pd1/1 -> Out1/1

== system gm_gmStateSpaceHDL_uz_inverter_3ph/uz_inverter_3ph/Data Type Conversion8 ==
  In1 : Inport
  Data Type Conversion8 : DataTypeConversion  OutDataTypeStr=double  RndMeth=Nearest  SampleTime=1e-08
  Data Type Conversion8_pd1 : Delay  DelayLength=3
  Out1 : Outport
  wires:
  In1/1 -> Data Type Conversion8/1
  Data Type Conversion8/1 -> Data Type Conversion8_pd1/1
  Data Type Conversion8_pd1/1 -> Out1/1

== system gm_gmStateSpaceHDL_uz_inverter_3ph/uz_inverter_3ph/Data Type Conversion9 ==
  In1 : Inport
  Data Type Conversion9 : DataTypeConversion  OutDataTypeStr=double  RndMeth=Nearest  SampleTime=1e-08
  Data Type Conversion9_pd1 : Delay  DelayLength=3
  Out1 : Outport
  wires:
  In1/1 -> Data Type Conversion9/1
  Data Type Conversion9/1 -> Data Type Conversion9_pd1/1
  Data Type Conversion9_pd1/1 -> Out1/1

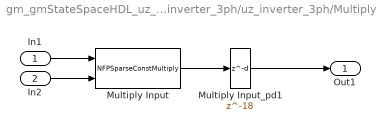
== system gm_gmStateSpaceHDL_uz_inverter_3ph/uz_inverter_3ph/Multiply Input ==
  In1 : Inport
  In2 : Inport  Port=2
  Multiply Input : hdlssclib/NFPSparseConstMultiply  constMatrix="reshape(single([-0.9999997615814209 -0.9999997615814209 -0.9999997615814209 -2.199999514160278e-12 2.1999994714860804e-05 -1.99999976757681e-05 1.99999976757681e-06 -2.199999514160278e-12 2.1999994714860804e-05 1.99999976757681e-06 2.1999994714860804e-05 1.99999976757681e-06 0 0 0 0 0 0 0 0 0 0 0 0 0 0 0 0 0 0 0 0 0 0 0 0 0 0 0 0 0 0 0 0 0 0 0 0 0 0 0 0 0 0 0 0 0 0 0 0 0 0 0 0 0 0 0 0 0 0 0 0 0 0 0 0 0 0 0 0 0 0 0 0 -0.009999997913837433 0 0.009999997913837433 9.999997985232767e-08 -0.9999997615814209 9.999997985232767e-08 -9.999998162868451e-09 0 0 9.999998162868451e-09 0.9999997615814209 0 0 -0.009999997913837433 0.009999997913837433 0 0 9.999997985232767e-08 -9.999998162868451e-09 9.999997985232767e-08 -0.9999997615814209 0 0.9999997615814209 9.999998162868451e-09 0.9999997615814209 -0.9999997615814209 -0.9999997615814209 -1.99999976757681e-05 1.99999976757681e-06 -1.99999976757681e-05 1.99999976757681e-06 -2.199999514160278e-12 2.1999994714860804e-05 2.1999994714860804e-05 2.1999994714860804e-05 1.99999976757681e-06 0 0 0 0 0 0 0 0 0 0 0 0 0 0 0 0 0 0 0 0 0 0 0 0 0 0 0 0 0 0 0 0 0 0 0 0 0 0 0 0 0 0 0 0 0 0 0 0 0 0 0 0 0 0 0 0 0 0 0 0 0 0 0 0 0 0 0 0 0 0 0 0 -0.009999997913837433 0 0.009999997913837433 9.999997985232767e-08 -9.999998162868451e-09 9.999997985232767e-08 -9.999998162868451e-09 0 0 0.9999997615814209 0.9999997615814209 0 0 -0.009999997913837433 0.009999997913837433 0 0 9.999997985232767e-08 -9.999998162868451e-09 9.999997985232767e-08 -0.9999997615814209 0 0.9999997615814209 9.999998162868451e-09 -0.9999997615814209 -0.9999997615814209 0.9999997615814209 -2.199999514160278e-12 2.1999994714860804e-05 -2.199999514160278e-12 2.1999994714860804e-05 -2.199999514160278e-12 2.1999994714860804e-05 1.99999976757681e-06 1.99999976757681e-06 1.99999976757681e-06 0 0 0 0 0 0 0 0 0 0 0 0 0 0 0 0 0 0 0 0 0 0 0 0 0 0 0 0 0 0 0 0 0 0 0 0 0 0 0 0 0 0 0 0 0 0 0 0 0 0 0 0 0 0 0 0 0 0 0 0 0 0 0 0 0 0 0 0 0 0 0 0 -0.009999997913837433 0 0.009999997913837433 9.999997985232767e-08 -0.9999997615814209 9.999997985232767e-08 -0.9999997615814209 0 0 9.999998162868451e-09 9.999998162868451e-09 0 0 -0.009999997913837433 0.009999997913837433 0 0 9.999997985232767e-08 -0.9999997615814209 9.999997985232767e-08 -0.9999997615814209 0 9.999998162868451e-09 9.999998162868451e-09 0.9999997615814209 -0.9999997615814209 0.9999997615814209 -1.99999976757681e-05 1.99999976757681e-06 -2.199999514160278e-12 2.1999994714860804e-05 -2.199999514160278e-12 2.1999994714860804e-05 2.1999994714860804e-05 1.99999976757681e-06 1.99999976757681e-06 0 0 0 0 0 0 0 0 0 0 0 0 0 0 0 0 0 0 0 0 0 0 0 0 0 0 0 0 0 0 0 0 0 0 0 0 0 0 0 0 0 0 0 0 0 0 0 0 0 0 0 0 0 0 0 0 0 0 0 0 0 0 0 0 0 0 0 0 0 0 0 0 -0.009999997913837433 0 0.009999997913837433 9.999997985232767e-08 -9.999998162868451e-09 9.999997985232767e-08 -0.9999997615814209 0 0 0.9999997615814209 9.999998162868451e-09 0 0 -0.009999997913837433 0.009999997913837433 0 0 9.999997985232767e-08 -0.9999997615814209 9.999997985232767e-08 -0.9999997615814209 0 9.999998162868451e-09 9.999998162868451e-09 -0.9999997615814209 0.9999997615814209 0.9999997615814209 -2.199999514160278e-12 2.1999994714860804e-05 -2.199999514160278e-12 2.1999994714860804e-05 -1.99999976757681e-05 1.99999976757681e-06 1.99999976757681e-06 1.99999976757681e-06 2.1999994714860804e-05 0 0 0 0 0 0 0 0 0 0 0 0 0 0 0 0 0 0 0 0 0 0 0 0 0 0 0 0 0 0 0 0 0 0 0 0 0 0 0 0 0 0 0 0 0 0 0 0 0 0 0 0 0 0 0 0 0 0 0 0 0 0 0 0 0 0 0 0 0 0 0 0 -0.009999997913837433 0 0.009999997913837433 9.999997985232767e-08 -0.9999997615814209 9.999997985232767e-08 -0.9999997615814209 0 0 9.999998162868451e-09 9.999998162868451e-09 0 0 -0.009999997913837433 0.009999997913837433 0 0 9.999997985232767e-08 -0.9999997615814209 9.999997985232767e-08 -9.999998162868451e-09 0 9.999998162868451e-09 0.9999997615814209 0.9999997615814209 0.9999997615814209 0.9999997615814209 -1.99999976757681e-05 1.99999976757681e-06 -2.199999514160278e-12 2.1999994714860804e-05 -1.99999976757681e-05 1.99999976757681e-06 ...(+2087 chars)]).', [12   9   8])"
      settings: SourceProductBaseCode=SL
  Multiply Input_pd1 : Delay  DelayLength=18
  Out1 : Outport
  wires:
  In1/1 -> Multiply Input/1
  In2/1 -> Multiply Input/2
  Multiply Input/1 -> Multiply Input_pd1/1
  Multiply Input_pd1/1 -> Out1/1

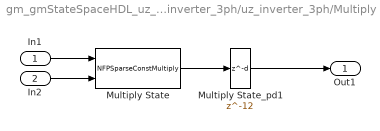
== system gm_gmStateSpaceHDL_uz_inverter_3ph/uz_inverter_3ph/Multiply State ==
  In1 : Inport
  In2 : Inport  Port=2
  Multiply State : hdlssclib/NFPSparseConstMultiply  constMatrix="reshape(single([1 0 -1 -1 1 0 0 -1 1 0 0 0 0 0 0 0 0 0 0 0 0 0 0 0 0 0 0 0 0 0 0 0 0 0 0 0]).', [3  12])"
      settings: SourceProductBaseCode=SL
  Multiply State_pd1 : Delay  DelayLength=12
  Out1 : Outport
  wires:
  In1/1 -> Multiply State/1
  In2/1 -> Multiply State/2
  Multiply State/1 -> Multiply State_pd1/1
  Multiply State_pd1/1 -> Out1/1
